simulink model "snap2_f_200msps_64i_4096c"  (R2019a)
settings: Solver=VariableStepDiscrete  StartTime=0.0  StopTime=10.0  RelTol=1e-3
undefined symbols (not defined in the file or in its folder): datetime, posixtime
libraries: xbsIndex_r4 x21354, casper_library_misc x297, casper_library_delays x19, xps_library x14, casper_library_sources x4
(part 40 of 217)

== system snap2_f_200msps_64i_4096c/pfb/pfb16x_0 ==
  note: reshape(reshape([0:8192 - 1], 16, 512)', 1, 8192)
  note: here we get a spectrum
      | 8 channels at a time. It takes
      | 512 clocks to get a full spectrum,
      | then we cycle through 16 inputs
  note: use 32 bit sync
      | because of bug
      | in blackboxing when
      | 1-bit inputs are used
  note: 16 parallel samples on each clock.
      | Consecutive clocks give next 16 samples
      | until all 8k have been sent (taking 512 clocks)
      | Then the block cycles through the different
      | pols
  note: 16 parallel samples on each clock cycle.
      | Consecutive clocks give:
      | pol0
      | pol1
      | ...
      | pol14
      | pol15
  note: Each output here
      | is a consecutive
      | samples for a single ADC
      | input
  note: use 32 bit sync
      | because of bug
      | in blackboxing when
      | 1-bit inputs are used
  sync : Inport
  fft_shift : Inport  Port=2
  din : Inport  Port=3
  stat_rst : Inport  Port=4
  skip_pfb : Inport  Port=5
  Constant : xbsIndex_r4/Constant  const=1.0  gui_display_data_type=Boolean  arith_type=Boolean  n_bits=16  bin_pt=14  preci_type=Single  exp_width=8  frac_width=24  explicit_period=on  period=1  equ=P=C  opselect=C  inp2=PCIN>>17  opr=+  inp1=P  carry=CIN  dbl_ovrd=off  block_type=constant
  Constant1 : xbsIndex_r4/Constant  const=0  gui_display_data_type=Fixed-point  arith_type=Unsigned  n_bits=16  bin_pt=0  preci_type=Single  exp_width=8  frac_width=24  explicit_period=on  period=1  equ=P=C  opselect=C  inp2=PCIN>>17  opr=+  inp1=P  carry=CIN  dbl_ovrd=off  block_type=constant
  Convert{,4..5,7..19} (16 alike) : xbsIndex_r4/Convert  gui_display_data_type=Fixed-point  arith_type="Signed  (2's comp)"  n_bits=18  bin_pt=17  float_type=Single  exp_bits=8  fraction_bits=24  quantization=Truncate  overflow=Wrap  en=off  latency=0  pipeline=off  dbl_ovrd=off  block_type=convert
  Convert1 : xbsIndex_r4/Convert  gui_display_data_type=Boolean  arith_type=Boolean  n_bits=16  bin_pt=0  float_type=Single  exp_bits=8  fraction_bits=24  quantization=Truncate  overflow=Wrap  en=off  latency=0  pipeline=off  dbl_ovrd=off  block_type=convert
  Convert2 : xbsIndex_r4/Convert  gui_display_data_type=Fixed-point  arith_type=Unsigned  n_bits=32  bin_pt=0  float_type=Single  exp_bits=8  fraction_bits=24  quantization=Truncate  overflow=Wrap  en=off  latency=0  pipeline=off  dbl_ovrd=off  block_type=convert
  Convert3 : xbsIndex_r4/Convert  gui_display_data_type=Boolean  arith_type=Boolean  n_bits=16  bin_pt=0  float_type=Single  exp_bits=8  fraction_bits=24  quantization=Truncate  overflow=Wrap  en=off  latency=0  pipeline=off  dbl_ovrd=off  block_type=convert
  Convert6 : xbsIndex_r4/Convert  gui_display_data_type=Fixed-point  arith_type=Unsigned  n_bits=32  bin_pt=0  float_type=Single  exp_bits=8  fraction_bits=24  quantization=Truncate  overflow=Wrap  en=off  latency=0  pipeline=off  dbl_ovrd=off  block_type=convert
  Delay : xbsIndex_r4/Delay  rst=off  infoeditControl=Selection of Reset will increase slice count due to use of real FFs and instead of SRLs  en=off  latency=1  reg_retiming=off  dbl_ovrd=off  block_type=delay
  Delay1 : xbsIndex_r4/Delay  rst=off  infoeditControl=Selection of Reset will increase slice count due to use of real FFs and instead of SRLs  en=off  latency=1  reg_retiming=off  dbl_ovrd=off  block_type=delay
  Mux : xbsIndex_r4/Mux  inputs=2  en=off  latency=1  precision=Full  arith_type=Unsigned  n_bits=16  bin_pt=14  quantization=Truncate  overflow=Wrap  dbl_ovrd=off  block_type=mux
  Mux1 : xbsIndex_r4/Mux  inputs=2  en=off  latency=1  precision=Full  arith_type=Unsigned  n_bits=16  bin_pt=14  quantization=Truncate  overflow=Wrap  dbl_ovrd=off  block_type=mux
  Relational : xbsIndex_r4/Relational  mode=a!=b  op_type=Bool  en=off  latency=1  dbl_ovrd=off  block_type=relational
  bus_create : Subsystem  AncestorBlock=casper_library_flow_control/bus_create  mask(bus_create){inputNum=16}
      mask prompts: inputNum "Number of inputs:"
      mask init:
      | bus_create_init(gcb,...
      |     'inputNum', inputNum);
  bus_create2 : Subsystem  AncestorBlock=casper_library_flow_control/bus_create  mask(bus_create){inputNum=16}
      mask prompts: inputNum "Number of inputs:"
      mask init:
      | bus_create_init(gcb,...
      |     'inputNum', inputNum);
  bus_expand : Subsystem  AncestorBlock=casper_library_flow_control/bus_expand  mask(bus_expand){mode=divisions of equal size, outputNum=16, outputWidth=10, outputBinaryPt=9, outputArithmeticType=1, show_format=off, outputToWorkspace=off, variablePrefix=out, outputToModelAsWell=on}
      mask prompts: outputNum "Number of outputs:"; outputWidth "Output width:"; outputBinaryPt "Output binary point position:"; outputArithmeticType "Output arithmetic type (ufix=0, fix=1, bool=2):"; show_format "Print format string?"; outputToWorkspace "Output to workspace?"; variablePrefix "Variable name prefix:"; outputToModelAsWell "Output to model as well?"
      mask help:
      | Expands a 'bus' made using a bus_create or Xilinx
      | concat block.
      | The input will be divided into the specified number
      | of outputs with the specified arithmetic types.
      | Divisions are made from most significant bit.
      mask init: same as snap2_f_200msps_64i_4096c/autocorr/bus_expand
      settings: AttributesFormatString=16 outputs
      mask TypeOptions mode: divisions of equal size | divisions of arbitrary size
      mask Callback mode: bus_expand_callback();
      mask Callback outputWidth: bus_expand_callback();
      mask Callback outputToWorkspace: bus_expand_callback();
  bus_expand4 : Subsystem  AncestorBlock=casper_library_flow_control/bus_expand  mask(bus_expand){mode=divisions of equal size, outputNum=16, outputWidth=10, outputBinaryPt=0, outputArithmeticType=0, show_format=off, outputToWorkspace=off, variablePrefix=out, outputToModelAsWell=on}
      mask prompts: outputNum "Number of outputs:"; outputWidth "Output width:"; outputBinaryPt "Output binary point position:"; outputArithmeticType "Output arithmetic type (ufix=0, fix=1, bool=2):"; show_format "Print format string?"; outputToWorkspace "Output to workspace?"; variablePrefix "Variable name prefix:"; outputToModelAsWell "Output to model as well?"
      mask help:
      | Expands a 'bus' made using a bus_create or Xilinx
      | concat block.
      | The input will be divided into the specified number
      | of outputs with the specified arithmetic types.
      | Divisions are made from most significant bit.
      mask init: same as snap2_f_200msps_64i_4096c/autocorr/bus_expand
      settings: AttributesFormatString=16 outputs
      mask TypeOptions mode: divisions of equal size | divisions of arbitrary size
      mask Callback mode: bus_expand_callback();
      mask Callback outputWidth: bus_expand_callback();
      mask Callback outputToWorkspace: bus_expand_callback();
  fft_4096_1i : xbsIndex_r4/Black Box  init_code=fft_4096c_1i_core_config  sim_method=Inactive  verbose=off  block_type=blackbox2
  of_count : xbsIndex_r4/Counter  cnt_type=Free Running  cnt_to=Inf  operation=Up  start_count=0  cnt_by_val=1  arith_type=Unsigned  n_bits=32  bin_pt=0  load_pin=off  rst=on  en=on  explicit_period=on  period=1  use_behavioral_HDL=off  implementation=DSP48  dbl_ovrd=off  block_type=counter
  pfb_fir_4096ch_bb : xbsIndex_r4/Black Box  init_code=pfb_fir_4096c_16i_core_config  sim_method=Inactive  verbose=off  block_type=blackbox2
  reorder1 : Subsystem  AncestorBlock=casper_library_reorder/reorder  mask(reorder){map=reshape(reshape([0:8192 - 1], 16, 512)', 1, 8192), n_bits=160, n_inputs=1, bram_latency=2, map_latency=2, fanout_latency=0, double_buffer=0, bram_map=on, software_controlled=off}
      mask prompts: map "Output Order:"; n_bits "Data width in"; n_inputs "Number of inputs"; bram_latency "BRAM Latency"; map_latency "Map Latency"; fanout_latency "Fanout latency"; double_buffer "Double Buffer"; bram_map "Use BlockRAM for Map"; software_controlled "Use runtime software control"
      mask init: same as snap2_f_200msps_64i_4096c/chan_reorder/dynamic
      settings: AttributesFormatString=order=13
      mask Help: eval('xlWeb(''http://casper.berkeley.edu/wiki/Reorder'')')
  square_transposer : Subsystem  AncestorBlock=casper_library_reorder/square_transposer  mask(square_transposer){n_inputs=4, async=off}
      mask prompts: n_inputs "Number of inputs (2^?):"; async "Aynchronus operation"
      mask init:
      | square_transposer_init(gcb,...
      |     'n_inputs', n_inputs, ...
      |     'async', async);
      settings: AttributesFormatString=n_inputs=4
      mask Help: eval('xlWeb(''http://casper.berkeley.edu/wiki/Square_transposer'')')
  status : Subsystem  Tag=xps:sw_reg  AncestorBlock=xps_library/Memory/software_register  mask(swreg){io_dir=To Processor, io_delay=0, init_val=0, sample_period=1, names=reg, bitwidths=32, bin_pts=0, arith_types=0, sim_port=on, show_format=off, desc_str=|}
      mask desc_str=|
      | A 32-bit counter which, for register name suffix
      | ``<n>_status`` increments every time an FFT
      | overflow event is detected in any of FFT channels
      | ``16n..16(n+1)-1``. Resets only when
      | commanded via the PFB control register, and will
      | wrap once the maximum value is reached.
      mask prompts: io_dir "I/O direction"; io_delay "I/O delay"; init_val "Initial Value"; sample_period "Sample period"; names "Bitfield names [msb...lsb]"; bitwidths "Bitfield widths"; bin_pts "Bitfield binary pts"; arith_types "Bitfield types, ufix=0, fix=1, bool=2"; sim_port "Provide sim input/output?"; show_format "Print format string?"; desc_str "Description"
      mask help: A 32-bit software-accessible register. Can be divided into bitfields of varying widths and types using the fields in the block mask.
      mask init:
      | swreg_init(gcb)
      settings: AttributesFormatString=1output
      mask TypeOptions io_dir: To Processor | From Processor
      mask Callback io_dir:
      | mask_enables = get_param(gcb, 'MaskEnables');
      | mask_names = get_param(gcb, 'MaskNames');
      | if strcmp(get_param(gcb, 'io_dir'), 'To Processor'),
      |     mask_enables{ismember(mask_names, 'sample_period')} = 'off';
      | else
      |     mask_enables{ismember(mask_names, 'sample_period')} = 'on';
      | end
      | set_param(gcb, 'MaskEnables', mask_enables);
      mask DialogControl ParameterTabVar0 Prompt: Setup
  sync_out : Outport
  dout : Outport  Port=2
  wires:
  bus_expand4/3(out14) -> square_transposer/4(in2)
  square_transposer/12(out10) -> bus_create2/11(in11)
  bus_expand4/16(lsb_out1) -> square_transposer/17(in15)
  bus_expand4/4(out13) -> square_transposer/5(in3)
  square_transposer/2(out0) -> bus_create2/1(in1)
  square_transposer/13(out11) -> bus_create2/12(in12)
  square_transposer/5(out3) -> bus_create2/4(in4)
  bus_expand4/2(out15) -> square_transposer/3(in1)
  square_transposer/16(out14) -> bus_create2/15(in15)
  bus_expand4/9(out8) -> square_transposer/10(in8)
  square_transposer/10(out8) -> bus_create2/9(in9)
  square_transposer/3(out1) -> bus_create2/2(in2)
  square_transposer/4(out2) -> bus_create2/3(in3)
  bus_expand4/8(out9) -> square_transposer/9(in7)
  square_transposer/15(out13) -> bus_create2/14(in14)
  bus_expand4/10(out7) -> square_transposer/11(in9)
  square_transposer/8(out6) -> bus_create2/7(in7)
  bus_expand4/13(out4) -> square_transposer/14(in12)
  square_transposer/11(out9) -> bus_create2/10(in10)
  bus_expand4/6(out11) -> square_transposer/7(in5)
  square_transposer/14(out12) -> bus_create2/13(in13)
  square_transposer/17(out15) -> bus_create2/16(in16)
  bus_expand4/12(out5) -> square_transposer/13(in11)
  square_transposer/6(out4) -> bus_create2/5(in5)
  square_transposer/7(out5) -> bus_create2/6(in6)
  bus_expand4/14(out3) -> square_transposer/15(in13)
  square_transposer/9(out7) -> bus_create2/8(in8)
  bus_expand4/15(out2) -> square_transposer/16(in14)
  bus_expand4/1(msb_out16) -> square_transposer/2(in0)
  bus_expand4/5(out12) -> square_transposer/6(in4)
  bus_expand4/7(out10) -> square_transposer/8(in6)
  bus_expand4/11(out6) -> square_transposer/12(in10)
  fft_shift/1 -> fft_4096_1i/2
  din/1 -> bus_expand4/1(bus_in)
  pfb_fir_4096ch_bb/1 -> Convert3/1
  fft_4096_1i/1 -> Convert1/1
  fft_4096_1i/2 -> dout/1
  Convert1/1 -> sync_out/1
  Convert2/1 -> pfb_fir_4096ch_bb/1
  Convert6/1 -> fft_4096_1i/1
  fft_4096_1i/3 -> Relational/1
  sync/1 -> square_transposer/1(sync)
  bus_create2/1(bus_out) -> reorder1/3(din0)
  square_transposer/1(sync_out) -> reorder1/1(sync)
  Constant/1 -> reorder1/2(en)
  reorder1/1(sync_out) -> Mux1/3, Convert2/1
  reorder1/3(dout0) -> pfb_fir_4096ch_bb/2, bus_expand/1(bus_in)
  of_count/1 -> status/1(out_reg)
  Constant1/1 -> Relational/2
  Relational/1 -> of_count/2
  stat_rst/1 -> of_count/1
  bus_expand/1(msb_out16) -> Convert/1
  bus_expand/3(out14) -> Convert5/1
  bus_expand/2(out15) -> Convert4/1
  bus_expand/4(out13) -> Convert7/1
  bus_expand/8(out9) -> Convert11/1
  bus_expand/6(out11) -> Convert9/1
  bus_expand/7(out10) -> Convert10/1
  bus_expand/5(out12) -> Convert8/1
  bus_expand/13(out4) -> Convert18/1
  bus_expand/15(out2) -> Convert13/1
  bus_expand/14(out3) -> Convert19/1
  bus_expand/16(lsb_out1) -> Convert14/1
  bus_expand/12(out5) -> Convert17/1
  bus_expand/10(out7) -> Convert15/1
  bus_expand/11(out6) -> Convert16/1
  bus_expand/9(out8) -> Convert12/1
  Convert/1 -> bus_create/1(in1)
  Convert4/1 -> bus_create/2(in2)
  Convert5/1 -> bus_create/3(in3)
  Convert7/1 -> bus_create/4(in4)
  Convert8/1 -> bus_create/5(in5)
  Convert9/1 -> bus_create/6(in6)
  Convert10/1 -> bus_create/7(in7)
  Convert11/1 -> bus_create/8(in8)
  Convert12/1 -> bus_create/9(in9)
  Convert15/1 -> bus_create/10(in10)
  Convert16/1 -> bus_create/11(in11)
  Convert17/1 -> bus_create/12(in12)
  Convert18/1 -> bus_create/13(in13)
  Convert19/1 -> bus_create/14(in14)
  Convert13/1 -> bus_create/15(in15)
  Convert14/1 -> bus_create/16(in16)
  pfb_fir_4096ch_bb/2 -> Mux/2
  bus_create/1(bus_out) -> Mux/3
  Delay/1 -> Mux/1
  Delay1/1 -> Mux1/1
  Convert3/1 -> Mux1/2
  skip_pfb/1 -> Delay/1, Delay1/1
  Mux1/1 -> Convert6/1
  Mux/1 -> fft_4096_1i/3

== system snap2_f_200msps_64i_4096c/pfb/pfb16x_1 ==
  note: use 32 bit sync
      | because of bug
      | in blackboxing when
      | 1-bit inputs are used
  note: Each output here
      | is a consecutive
      | samples for a single ADC
      | input
  note: 16 parallel samples on each clock cycle.
      | Consecutive clocks give:
      | pol0
      | pol1
      | ...
      | pol14
      | pol15
  note: 16 parallel samples on each clock.
      | Consecutive clocks give next 16 samples
      | until all 8k have been sent (taking 512 clocks)
      | Then the block cycles through the different
      | pols
  note: use 32 bit sync
      | because of bug
      | in blackboxing when
      | 1-bit inputs are used
  note: here we get a spectrum
      | 8 channels at a time. It takes
      | 512 clocks to get a full spectrum,
      | then we cycle through 16 inputs
  note: reshape(reshape([0:8192 - 1], 16, 512)', 1, 8192)
  sync : Inport
  fft_shift : Inport  Port=2
  din : Inport  Port=3
  stat_rst : Inport  Port=4
  skip_pfb : Inport  Port=5
  Constant : xbsIndex_r4/Constant  const=1.0  gui_display_data_type=Boolean  arith_type=Boolean  n_bits=16  bin_pt=14  preci_type=Single  exp_width=8  frac_width=24  explicit_period=on  period=1  equ=P=C  opselect=C  inp2=PCIN>>17  opr=+  inp1=P  carry=CIN  dbl_ovrd=off  block_type=constant
  Constant1 : xbsIndex_r4/Constant  const=0  gui_display_data_type=Fixed-point  arith_type=Unsigned  n_bits=16  bin_pt=0  preci_type=Single  exp_width=8  frac_width=24  explicit_period=on  period=1  equ=P=C  opselect=C  inp2=PCIN>>17  opr=+  inp1=P  carry=CIN  dbl_ovrd=off  block_type=constant
  Convert{,4..5,7..19} (16 alike) : xbsIndex_r4/Convert  gui_display_data_type=Fixed-point  arith_type="Signed  (2's comp)"  n_bits=18  bin_pt=17  float_type=Single  exp_bits=8  fraction_bits=24  quantization=Truncate  overflow=Wrap  en=off  latency=0  pipeline=off  dbl_ovrd=off  block_type=convert
  Convert1 : xbsIndex_r4/Convert  gui_display_data_type=Boolean  arith_type=Boolean  n_bits=16  bin_pt=0  float_type=Single  exp_bits=8  fraction_bits=24  quantization=Truncate  overflow=Wrap  en=off  latency=0  pipeline=off  dbl_ovrd=off  block_type=convert
  Convert2 : xbsIndex_r4/Convert  gui_display_data_type=Fixed-point  arith_type=Unsigned  n_bits=32  bin_pt=0  float_type=Single  exp_bits=8  fraction_bits=24  quantization=Truncate  overflow=Wrap  en=off  latency=0  pipeline=off  dbl_ovrd=off  block_type=convert
  Convert3 : xbsIndex_r4/Convert  gui_display_data_type=Boolean  arith_type=Boolean  n_bits=16  bin_pt=0  float_type=Single  exp_bits=8  fraction_bits=24  quantization=Truncate  overflow=Wrap  en=off  latency=0  pipeline=off  dbl_ovrd=off  block_type=convert
  Convert6 : xbsIndex_r4/Convert  gui_display_data_type=Fixed-point  arith_type=Unsigned  n_bits=32  bin_pt=0  float_type=Single  exp_bits=8  fraction_bits=24  quantization=Truncate  overflow=Wrap  en=off  latency=0  pipeline=off  dbl_ovrd=off  block_type=convert
  Delay : xbsIndex_r4/Delay  rst=off  infoeditControl=Selection of Reset will increase slice count due to use of real FFs and instead of SRLs  en=off  latency=1  reg_retiming=off  dbl_ovrd=off  block_type=delay
  Delay1 : xbsIndex_r4/Delay  rst=off  infoeditControl=Selection of Reset will increase slice count due to use of real FFs and instead of SRLs  en=off  latency=1  reg_retiming=off  dbl_ovrd=off  block_type=delay
  Mux : xbsIndex_r4/Mux  inputs=2  en=off  latency=1  precision=Full  arith_type=Unsigned  n_bits=16  bin_pt=14  quantization=Truncate  overflow=Wrap  dbl_ovrd=off  block_type=mux
  Mux1 : xbsIndex_r4/Mux  inputs=2  en=off  latency=1  precision=Full  arith_type=Unsigned  n_bits=16  bin_pt=14  quantization=Truncate  overflow=Wrap  dbl_ovrd=off  block_type=mux
  Relational : xbsIndex_r4/Relational  mode=a!=b  op_type=Bool  en=off  latency=1  dbl_ovrd=off  block_type=relational
  bus_create : Subsystem  AncestorBlock=casper_library_flow_control/bus_create  mask(bus_create){inputNum=16}
      mask prompts: inputNum "Number of inputs:"
      mask init:
      | bus_create_init(gcb,...
      |     'inputNum', inputNum);
  bus_create2 : Subsystem  AncestorBlock=casper_library_flow_control/bus_create  mask(bus_create){inputNum=16}
      mask prompts: inputNum "Number of inputs:"
      mask init:
      | bus_create_init(gcb,...
      |     'inputNum', inputNum);
  bus_expand : Subsystem  AncestorBlock=casper_library_flow_control/bus_expand  mask(bus_expand){mode=divisions of equal size, outputNum=16, outputWidth=10, outputBinaryPt=9, outputArithmeticType=1, show_format=off, outputToWorkspace=off, variablePrefix=out, outputToModelAsWell=on}
      mask prompts: outputNum "Number of outputs:"; outputWidth "Output width:"; outputBinaryPt "Output binary point position:"; outputArithmeticType "Output arithmetic type (ufix=0, fix=1, bool=2):"; show_format "Print format string?"; outputToWorkspace "Output to workspace?"; variablePrefix "Variable name prefix:"; outputToModelAsWell "Output to model as well?"
      mask help:
      | Expands a 'bus' made using a bus_create or Xilinx
      | concat block.
      | The input will be divided into the specified number
      | of outputs with the specified arithmetic types.
      | Divisions are made from most significant bit.
      mask init: same as snap2_f_200msps_64i_4096c/autocorr/bus_expand
      settings: AttributesFormatString=16 outputs
      mask TypeOptions mode: divisions of equal size | divisions of arbitrary size
      mask Callback mode: bus_expand_callback();
      mask Callback outputWidth: bus_expand_callback();
      mask Callback outputToWorkspace: bus_expand_callback();
  bus_expand4 : Subsystem  AncestorBlock=casper_library_flow_control/bus_expand  mask(bus_expand){mode=divisions of equal size, outputNum=16, outputWidth=10, outputBinaryPt=0, outputArithmeticType=0, show_format=off, outputToWorkspace=off, variablePrefix=out, outputToModelAsWell=on}
      mask prompts: outputNum "Number of outputs:"; outputWidth "Output width:"; outputBinaryPt "Output binary point position:"; outputArithmeticType "Output arithmetic type (ufix=0, fix=1, bool=2):"; show_format "Print format string?"; outputToWorkspace "Output to workspace?"; variablePrefix "Variable name prefix:"; outputToModelAsWell "Output to model as well?"
      mask help:
      | Expands a 'bus' made using a bus_create or Xilinx
      | concat block.
      | The input will be divided into the specified number
      | of outputs with the specified arithmetic types.
      | Divisions are made from most significant bit.
      mask init: same as snap2_f_200msps_64i_4096c/autocorr/bus_expand
      settings: AttributesFormatString=16 outputs
      mask TypeOptions mode: divisions of equal size | divisions of arbitrary size
      mask Callback mode: bus_expand_callback();
      mask Callback outputWidth: bus_expand_callback();
      mask Callback outputToWorkspace: bus_expand_callback();
  fft_4096_1i : xbsIndex_r4/Black Box  init_code=fft_4096c_1i_core_config  sim_method=Inactive  verbose=off  block_type=blackbox2
  of_count : xbsIndex_r4/Counter  cnt_type=Free Running  cnt_to=Inf  operation=Up  start_count=0  cnt_by_val=1  arith_type=Unsigned  n_bits=32  bin_pt=0  load_pin=off  rst=on  en=on  explicit_period=on  period=1  use_behavioral_HDL=off  implementation=DSP48  dbl_ovrd=off  block_type=counter
  pfb_fir_4096ch_bb : xbsIndex_r4/Black Box  init_code=pfb_fir_4096c_16i_core_config  sim_method=Inactive  verbose=off  block_type=blackbox2
  reorder1 : Subsystem  AncestorBlock=casper_library_reorder/reorder  mask(reorder){map=reshape(reshape([0:8192 - 1], 16, 512)', 1, 8192), n_bits=160, n_inputs=1, bram_latency=2, map_latency=2, fanout_latency=0, double_buffer=0, bram_map=on, software_controlled=off}
      mask prompts: map "Output Order:"; n_bits "Data width in"; n_inputs "Number of inputs"; bram_latency "BRAM Latency"; map_latency "Map Latency"; fanout_latency "Fanout latency"; double_buffer "Double Buffer"; bram_map "Use BlockRAM for Map"; software_controlled "Use runtime software control"
      mask init: same as snap2_f_200msps_64i_4096c/chan_reorder/dynamic
      settings: AttributesFormatString=order=13
      mask Help: eval('xlWeb(''http://casper.berkeley.edu/wiki/Reorder'')')
  square_transposer : Subsystem  AncestorBlock=casper_library_reorder/square_transposer  mask(square_transposer){n_inputs=4, async=off}
      mask prompts: n_inputs "Number of inputs (2^?):"; async "Aynchronus operation"
      mask init:
      | square_transposer_init(gcb,...
      |     'n_inputs', n_inputs, ...
      |     'async', async);
      settings: AttributesFormatString=n_inputs=4
      mask Help: eval('xlWeb(''http://casper.berkeley.edu/wiki/Square_transposer'')')
  status : Subsystem  Tag=xps:sw_reg  AncestorBlock=xps_library/Memory/software_register  mask(swreg){io_dir=To Processor, io_delay=0, init_val=0, sample_period=1, names=reg, bitwidths=32, bin_pts=0, arith_types=0, sim_port=on, show_format=off, desc_str=|}
      mask desc_str=|
      | A 32-bit counter which, for register name suffix
      | ``<n>_status`` increments every time an FFT
      | overflow event is detected in any of FFT channels
      | ``16n..16(n+1)-1``. Resets only when
      | commanded via the PFB control register, and will
      | wrap once the maximum value is reached.
      mask prompts: io_dir "I/O direction"; io_delay "I/O delay"; init_val "Initial Value"; sample_period "Sample period"; names "Bitfield names [msb...lsb]"; bitwidths "Bitfield widths"; bin_pts "Bitfield binary pts"; arith_types "Bitfield types, ufix=0, fix=1, bool=2"; sim_port "Provide sim input/output?"; show_format "Print format string?"; desc_str "Description"
      mask help: A 32-bit software-accessible register. Can be divided into bitfields of varying widths and types using the fields in the block mask.
      mask init:
      | swreg_init(gcb)
      settings: AttributesFormatString=1output
      mask TypeOptions io_dir: To Processor | From Processor
      mask Callback io_dir:
      | mask_enables = get_param(gcb, 'MaskEnables');
      | mask_names = get_param(gcb, 'MaskNames');
      | if strcmp(get_param(gcb, 'io_dir'), 'To Processor'),
      |     mask_enables{ismember(mask_names, 'sample_period')} = 'off';
      | else
      |     mask_enables{ismember(mask_names, 'sample_period')} = 'on';
      | end
      | set_param(gcb, 'MaskEnables', mask_enables);
      mask DialogControl ParameterTabVar0 Prompt: Setup
  sync_out : Outport
  dout : Outport  Port=2
  wires:
  Mux/1 -> fft_4096_1i/3
  Mux1/1 -> Convert6/1
  skip_pfb/1 -> Delay1/1, Delay/1
  Convert3/1 -> Mux1/2
  Delay1/1 -> Mux1/1
  Delay/1 -> Mux/1
  bus_create/1(bus_out) -> Mux/3
  pfb_fir_4096ch_bb/2 -> Mux/2
  Convert14/1 -> bus_create/16(in16)
  Convert13/1 -> bus_create/15(in15)
  Convert19/1 -> bus_create/14(in14)
  Convert18/1 -> bus_create/13(in13)
  Convert17/1 -> bus_create/12(in12)
  Convert16/1 -> bus_create/11(in11)
  Convert15/1 -> bus_create/10(in10)
  Convert12/1 -> bus_create/9(in9)
  Convert11/1 -> bus_create/8(in8)
  Convert10/1 -> bus_create/7(in7)
  Convert9/1 -> bus_create/6(in6)
  Convert8/1 -> bus_create/5(in5)
  Convert7/1 -> bus_create/4(in4)
  Convert5/1 -> bus_create/3(in3)
  Convert4/1 -> bus_create/2(in2)
  Convert/1 -> bus_create/1(in1)
  bus_expand/9(out8) -> Convert12/1
  bus_expand/11(out6) -> Convert16/1
  bus_expand/10(out7) -> Convert15/1
  bus_expand/12(out5) -> Convert17/1
  bus_expand/16(lsb_out1) -> Convert14/1
  bus_expand/14(out3) -> Convert19/1
  bus_expand/15(out2) -> Convert13/1
  bus_expand/13(out4) -> Convert18/1
  bus_expand/5(out12) -> Convert8/1
  bus_expand/7(out10) -> Convert10/1
  bus_expand/6(out11) -> Convert9/1
  bus_expand/8(out9) -> Convert11/1
  bus_expand/4(out13) -> Convert7/1
  bus_expand/2(out15) -> Convert4/1
  bus_expand/3(out14) -> Convert5/1
  bus_expand/1(msb_out16) -> Convert/1
  stat_rst/1 -> of_count/1
  Relational/1 -> of_count/2
  Constant1/1 -> Relational/2
  of_count/1 -> status/1(out_reg)
  reorder1/3(dout0) -> bus_expand/1(bus_in), pfb_fir_4096ch_bb/2
  reorder1/1(sync_out) -> Convert2/1, Mux1/3
  Constant/1 -> reorder1/2(en)
  square_transposer/1(sync_out) -> reorder1/1(sync)
  bus_create2/1(bus_out) -> reorder1/3(din0)
  sync/1 -> square_transposer/1(sync)
  fft_4096_1i/3 -> Relational/1
  Convert6/1 -> fft_4096_1i/1
  Convert2/1 -> pfb_fir_4096ch_bb/1
  Convert1/1 -> sync_out/1
  fft_4096_1i/2 -> dout/1
  fft_4096_1i/1 -> Convert1/1
  pfb_fir_4096ch_bb/1 -> Convert3/1
  din/1 -> bus_expand4/1(bus_in)
  fft_shift/1 -> fft_4096_1i/2
  bus_expand4/11(out6) -> square_transposer/12(in10)
  bus_expand4/7(out10) -> square_transposer/8(in6)
  bus_expand4/5(out12) -> square_transposer/6(in4)
  bus_expand4/1(msb_out16) -> square_transposer/2(in0)
  bus_expand4/15(out2) -> square_transposer/16(in14)
  square_transposer/9(out7) -> bus_create2/8(in8)
  bus_expand4/14(out3) -> square_transposer/15(in13)
  square_transposer/7(out5) -> bus_create2/6(in6)
  square_transposer/6(out4) -> bus_create2/5(in5)
  bus_expand4/12(out5) -> square_transposer/13(in11)
  square_transposer/17(out15) -> bus_create2/16(in16)
  square_transposer/14(out12) -> bus_create2/13(in13)
  bus_expand4/6(out11) -> square_transposer/7(in5)
  square_transposer/11(out9) -> bus_create2/10(in10)
  bus_expand4/13(out4) -> square_transposer/14(in12)
  square_transposer/8(out6) -> bus_create2/7(in7)
  bus_expand4/10(out7) -> square_transposer/11(in9)
  square_transposer/15(out13) -> bus_create2/14(in14)
  bus_expand4/8(out9) -> square_transposer/9(in7)
  square_transposer/4(out2) -> bus_create2/3(in3)
  square_transposer/3(out1) -> bus_create2/2(in2)
  square_transposer/10(out8) -> bus_create2/9(in9)
  bus_expand4/9(out8) -> square_transposer/10(in8)
  square_transposer/16(out14) -> bus_create2/15(in15)
  bus_expand4/2(out15) -> square_transposer/3(in1)
  square_transposer/5(out3) -> bus_create2/4(in4)
  square_transposer/13(out11) -> bus_create2/12(in12)
  square_transposer/2(out0) -> bus_create2/1(in1)
  bus_expand4/4(out13) -> square_transposer/5(in3)
  bus_expand4/16(lsb_out1) -> square_transposer/17(in15)
  square_transposer/12(out10) -> bus_create2/11(in11)
  bus_expand4/3(out14) -> square_transposer/4(in2)

== system snap2_f_200msps_64i_4096c/pfb/pfb16x_2 ==
  note: reshape(reshape([0:8192 - 1], 16, 512)', 1, 8192)
  note: here we get a spectrum
      | 8 channels at a time. It takes
      | 512 clocks to get a full spectrum,
      | then we cycle through 16 inputs
  note: use 32 bit sync
      | because of bug
      | in blackboxing when
      | 1-bit inputs are used
  note: 16 parallel samples on each clock.
      | Consecutive clocks give next 16 samples
      | until all 8k have been sent (taking 512 clocks)
      | Then the block cycles through the different
      | pols
  note: 16 parallel samples on each clock cycle.
      | Consecutive clocks give:
      | pol0
      | pol1
      | ...
      | pol14
      | pol15
  note: Each output here
      | is a consecutive
      | samples for a single ADC
      | input
  note: use 32 bit sync
      | because of bug
      | in blackboxing when
      | 1-bit inputs are used
  sync : Inport
  fft_shift : Inport  Port=2
  din : Inport  Port=3
  stat_rst : Inport  Port=4
  skip_pfb : Inport  Port=5
  Constant : xbsIndex_r4/Constant  const=1.0  gui_display_data_type=Boolean  arith_type=Boolean  n_bits=16  bin_pt=14  preci_type=Single  exp_width=8  frac_width=24  explicit_period=on  period=1  equ=P=C  opselect=C  inp2=PCIN>>17  opr=+  inp1=P  carry=CIN  dbl_ovrd=off  block_type=constant
  Constant1 : xbsIndex_r4/Constant  const=0  gui_display_data_type=Fixed-point  arith_type=Unsigned  n_bits=16  bin_pt=0  preci_type=Single  exp_width=8  frac_width=24  explicit_period=on  period=1  equ=P=C  opselect=C  inp2=PCIN>>17  opr=+  inp1=P  carry=CIN  dbl_ovrd=off  block_type=constant
  Convert{,4..5,7..19} (16 alike) : xbsIndex_r4/Convert  gui_display_data_type=Fixed-point  arith_type="Signed  (2's comp)"  n_bits=18  bin_pt=17  float_type=Single  exp_bits=8  fraction_bits=24  quantization=Truncate  overflow=Wrap  en=off  latency=0  pipeline=off  dbl_ovrd=off  block_type=convert
  Convert1 : xbsIndex_r4/Convert  gui_display_data_type=Boolean  arith_type=Boolean  n_bits=16  bin_pt=0  float_type=Single  exp_bits=8  fraction_bits=24  quantization=Truncate  overflow=Wrap  en=off  latency=0  pipeline=off  dbl_ovrd=off  block_type=convert
  Convert2 : xbsIndex_r4/Convert  gui_display_data_type=Fixed-point  arith_type=Unsigned  n_bits=32  bin_pt=0  float_type=Single  exp_bits=8  fraction_bits=24  quantization=Truncate  overflow=Wrap  en=off  latency=0  pipeline=off  dbl_ovrd=off  block_type=convert
  Convert3 : xbsIndex_r4/Convert  gui_display_data_type=Boolean  arith_type=Boolean  n_bits=16  bin_pt=0  float_type=Single  exp_bits=8  fraction_bits=24  quantization=Truncate  overflow=Wrap  en=off  latency=0  pipeline=off  dbl_ovrd=off  block_type=convert
  Convert6 : xbsIndex_r4/Convert  gui_display_data_type=Fixed-point  arith_type=Unsigned  n_bits=32  bin_pt=0  float_type=Single  exp_bits=8  fraction_bits=24  quantization=Truncate  overflow=Wrap  en=off  latency=0  pipeline=off  dbl_ovrd=off  block_type=convert
  Delay : xbsIndex_r4/Delay  rst=off  infoeditControl=Selection of Reset will increase slice count due to use of real FFs and instead of SRLs  en=off  latency=1  reg_retiming=off  dbl_ovrd=off  block_type=delay
  Delay1 : xbsIndex_r4/Delay  rst=off  infoeditControl=Selection of Reset will increase slice count due to use of real FFs and instead of SRLs  en=off  latency=1  reg_retiming=off  dbl_ovrd=off  block_type=delay
  Mux : xbsIndex_r4/Mux  inputs=2  en=off  latency=1  precision=Full  arith_type=Unsigned  n_bits=16  bin_pt=14  quantization=Truncate  overflow=Wrap  dbl_ovrd=off  block_type=mux
  Mux1 : xbsIndex_r4/Mux  inputs=2  en=off  latency=1  precision=Full  arith_type=Unsigned  n_bits=16  bin_pt=14  quantization=Truncate  overflow=Wrap  dbl_ovrd=off  block_type=mux
  Relational : xbsIndex_r4/Relational  mode=a!=b  op_type=Bool  en=off  latency=1  dbl_ovrd=off  block_type=relational
  bus_create : Subsystem  AncestorBlock=casper_library_flow_control/bus_create  mask(bus_create){inputNum=16}
      mask prompts: inputNum "Number of inputs:"
      mask init:
      | bus_create_init(gcb,...
      |     'inputNum', inputNum);
  bus_create2 : Subsystem  AncestorBlock=casper_library_flow_control/bus_create  mask(bus_create){inputNum=16}
      mask prompts: inputNum "Number of inputs:"
      mask init:
      | bus_create_init(gcb,...
      |     'inputNum', inputNum);
  bus_expand : Subsystem  AncestorBlock=casper_library_flow_control/bus_expand  mask(bus_expand){mode=divisions of equal size, outputNum=16, outputWidth=10, outputBinaryPt=9, outputArithmeticType=1, show_format=off, outputToWorkspace=off, variablePrefix=out, outputToModelAsWell=on}
      mask prompts: outputNum "Number of outputs:"; outputWidth "Output width:"; outputBinaryPt "Output binary point position:"; outputArithmeticType "Output arithmetic type (ufix=0, fix=1, bool=2):"; show_format "Print format string?"; outputToWorkspace "Output to workspace?"; variablePrefix "Variable name prefix:"; outputToModelAsWell "Output to model as well?"
      mask help:
      | Expands a 'bus' made using a bus_create or Xilinx
      | concat block.
      | The input will be divided into the specified number
      | of outputs with the specified arithmetic types.
      | Divisions are made from most significant bit.
      mask init: same as snap2_f_200msps_64i_4096c/autocorr/bus_expand
      settings: AttributesFormatString=16 outputs
      mask TypeOptions mode: divisions of equal size | divisions of arbitrary size
      mask Callback mode: bus_expand_callback();
      mask Callback outputWidth: bus_expand_callback();
      mask Callback outputToWorkspace: bus_expand_callback();
  bus_expand4 : Subsystem  AncestorBlock=casper_library_flow_control/bus_expand  mask(bus_expand){mode=divisions of equal size, outputNum=16, outputWidth=10, outputBinaryPt=0, outputArithmeticType=0, show_format=off, outputToWorkspace=off, variablePrefix=out, outputToModelAsWell=on}
      mask prompts: outputNum "Number of outputs:"; outputWidth "Output width:"; outputBinaryPt "Output binary point position:"; outputArithmeticType "Output arithmetic type (ufix=0, fix=1, bool=2):"; show_format "Print format string?"; outputToWorkspace "Output to workspace?"; variablePrefix "Variable name prefix:"; outputToModelAsWell "Output to model as well?"
      mask help:
      | Expands a 'bus' made using a bus_create or Xilinx
      | concat block.
      | The input will be divided into the specified number
      | of outputs with the specified arithmetic types.
      | Divisions are made from most significant bit.
      mask init: same as snap2_f_200msps_64i_4096c/autocorr/bus_expand
      settings: AttributesFormatString=16 outputs
      mask TypeOptions mode: divisions of equal size | divisions of arbitrary size
      mask Callback mode: bus_expand_callback();
      mask Callback outputWidth: bus_expand_callback();
      mask Callback outputToWorkspace: bus_expand_callback();
  fft_4096_1i : xbsIndex_r4/Black Box  init_code=fft_4096c_1i_core_config  sim_method=Inactive  verbose=off  block_type=blackbox2
  of_count : xbsIndex_r4/Counter  cnt_type=Free Running  cnt_to=Inf  operation=Up  start_count=0  cnt_by_val=1  arith_type=Unsigned  n_bits=32  bin_pt=0  load_pin=off  rst=on  en=on  explicit_period=on  period=1  use_behavioral_HDL=off  implementation=DSP48  dbl_ovrd=off  block_type=counter
  pfb_fir_4096ch_bb : xbsIndex_r4/Black Box  init_code=pfb_fir_4096c_16i_core_config  sim_method=Inactive  verbose=off  block_type=blackbox2
  reorder1 : Subsystem  AncestorBlock=casper_library_reorder/reorder  mask(reorder){map=reshape(reshape([0:8192 - 1], 16, 512)', 1, 8192), n_bits=160, n_inputs=1, bram_latency=2, map_latency=2, fanout_latency=0, double_buffer=0, bram_map=on, software_controlled=off}
      mask prompts: map "Output Order:"; n_bits "Data width in"; n_inputs "Number of inputs"; bram_latency "BRAM Latency"; map_latency "Map Latency"; fanout_latency "Fanout latency"; double_buffer "Double Buffer"; bram_map "Use BlockRAM for Map"; software_controlled "Use runtime software control"
      mask init: same as snap2_f_200msps_64i_4096c/chan_reorder/dynamic
      settings: AttributesFormatString=order=13
      mask Help: eval('xlWeb(''http://casper.berkeley.edu/wiki/Reorder'')')
  square_transposer : Subsystem  AncestorBlock=casper_library_reorder/square_transposer  mask(square_transposer){n_inputs=4, async=off}
      mask prompts: n_inputs "Number of inputs (2^?):"; async "Aynchronus operation"
      mask init:
      | square_transposer_init(gcb,...
      |     'n_inputs', n_inputs, ...
      |     'async', async);
      settings: AttributesFormatString=n_inputs=4
      mask Help: eval('xlWeb(''http://casper.berkeley.edu/wiki/Square_transposer'')')
  status : Subsystem  Tag=xps:sw_reg  AncestorBlock=xps_library/Memory/software_register  mask(swreg){io_dir=To Processor, io_delay=0, init_val=0, sample_period=1, names=reg, bitwidths=32, bin_pts=0, arith_types=0, sim_port=on, show_format=off, desc_str=|}
      mask desc_str=|
      | A 32-bit counter which, for register name suffix
      | ``<n>_status`` increments every time an FFT
      | overflow event is detected in any of FFT channels
      | ``16n..16(n+1)-1``. Resets only when
      | commanded via the PFB control register, and will
      | wrap once the maximum value is reached.
      mask prompts: io_dir "I/O direction"; io_delay "I/O delay"; init_val "Initial Value"; sample_period "Sample period"; names "Bitfield names [msb...lsb]"; bitwidths "Bitfield widths"; bin_pts "Bitfield binary pts"; arith_types "Bitfield types, ufix=0, fix=1, bool=2"; sim_port "Provide sim input/output?"; show_format "Print format string?"; desc_str "Description"
      mask help: A 32-bit software-accessible register. Can be divided into bitfields of varying widths and types using the fields in the block mask.
      mask init:
      | swreg_init(gcb)
      settings: AttributesFormatString=1output
      mask TypeOptions io_dir: To Processor | From Processor
      mask Callback io_dir:
      | mask_enables = get_param(gcb, 'MaskEnables');
      | mask_names = get_param(gcb, 'MaskNames');
      | if strcmp(get_param(gcb, 'io_dir'), 'To Processor'),
      |     mask_enables{ismember(mask_names, 'sample_period')} = 'off';
      | else
      |     mask_enables{ismember(mask_names, 'sample_period')} = 'on';
      | end
      | set_param(gcb, 'MaskEnables', mask_enables);
      mask DialogControl ParameterTabVar0 Prompt: Setup
  sync_out : Outport
  dout : Outport  Port=2
  wires:
  bus_expand4/3(out14) -> square_transposer/4(in2)
  square_transposer/12(out10) -> bus_create2/11(in11)
  bus_expand4/16(lsb_out1) -> square_transposer/17(in15)
  bus_expand4/4(out13) -> square_transposer/5(in3)
  square_transposer/2(out0) -> bus_create2/1(in1)
  square_transposer/13(out11) -> bus_create2/12(in12)
  square_transposer/5(out3) -> bus_create2/4(in4)
  bus_expand4/2(out15) -> square_transposer/3(in1)
  square_transposer/16(out14) -> bus_create2/15(in15)
  bus_expand4/9(out8) -> square_transposer/10(in8)
  square_transposer/10(out8) -> bus_create2/9(in9)
  square_transposer/3(out1) -> bus_create2/2(in2)
  square_transposer/4(out2) -> bus_create2/3(in3)
  bus_expand4/8(out9) -> square_transposer/9(in7)
  square_transposer/15(out13) -> bus_create2/14(in14)
  bus_expand4/10(out7) -> square_transposer/11(in9)
  square_transposer/8(out6) -> bus_create2/7(in7)
  bus_expand4/13(out4) -> square_transposer/14(in12)
  square_transposer/11(out9) -> bus_create2/10(in10)
  bus_expand4/6(out11) -> square_transposer/7(in5)
  square_transposer/14(out12) -> bus_create2/13(in13)
  square_transposer/17(out15) -> bus_create2/16(in16)
  bus_expand4/12(out5) -> square_transposer/13(in11)
  square_transposer/6(out4) -> bus_create2/5(in5)
  square_transposer/7(out5) -> bus_create2/6(in6)
  bus_expand4/14(out3) -> square_transposer/15(in13)
  square_transposer/9(out7) -> bus_create2/8(in8)
  bus_expand4/15(out2) -> square_transposer/16(in14)
  bus_expand4/1(msb_out16) -> square_transposer/2(in0)
  bus_expand4/5(out12) -> square_transposer/6(in4)
  bus_expand4/7(out10) -> square_transposer/8(in6)
  bus_expand4/11(out6) -> square_transposer/12(in10)
  fft_shift/1 -> fft_4096_1i/2
  din/1 -> bus_expand4/1(bus_in)
  pfb_fir_4096ch_bb/1 -> Convert3/1
  fft_4096_1i/1 -> Convert1/1
  fft_4096_1i/2 -> dout/1
  Convert1/1 -> sync_out/1
  Convert2/1 -> pfb_fir_4096ch_bb/1
  Convert6/1 -> fft_4096_1i/1
  fft_4096_1i/3 -> Relational/1
  sync/1 -> square_transposer/1(sync)
  bus_create2/1(bus_out) -> reorder1/3(din0)
  square_transposer/1(sync_out) -> reorder1/1(sync)
  Constant/1 -> reorder1/2(en)
  reorder1/1(sync_out) -> Mux1/3, Convert2/1
  reorder1/3(dout0) -> pfb_fir_4096ch_bb/2, bus_expand/1(bus_in)
  of_count/1 -> status/1(out_reg)
  Constant1/1 -> Relational/2
  Relational/1 -> of_count/2
  stat_rst/1 -> of_count/1
  bus_expand/1(msb_out16) -> Convert/1
  bus_expand/3(out14) -> Convert5/1
  bus_expand/2(out15) -> Convert4/1
  bus_expand/4(out13) -> Convert7/1
  bus_expand/8(out9) -> Convert11/1
  bus_expand/6(out11) -> Convert9/1
  bus_expand/7(out10) -> Convert10/1
  bus_expand/5(out12) -> Convert8/1
  bus_expand/13(out4) -> Convert18/1
  bus_expand/15(out2) -> Convert13/1
  bus_expand/14(out3) -> Convert19/1
  bus_expand/16(lsb_out1) -> Convert14/1
  bus_expand/12(out5) -> Convert17/1
  bus_expand/10(out7) -> Convert15/1
  bus_expand/11(out6) -> Convert16/1
  bus_expand/9(out8) -> Convert12/1
  Convert/1 -> bus_create/1(in1)
  Convert4/1 -> bus_create/2(in2)
  Convert5/1 -> bus_create/3(in3)
  Convert7/1 -> bus_create/4(in4)
  Convert8/1 -> bus_create/5(in5)
  Convert9/1 -> bus_create/6(in6)
  Convert10/1 -> bus_create/7(in7)
  Convert11/1 -> bus_create/8(in8)
  Convert12/1 -> bus_create/9(in9)
  Convert15/1 -> bus_create/10(in10)
  Convert16/1 -> bus_create/11(in11)
  Convert17/1 -> bus_create/12(in12)
  Convert18/1 -> bus_create/13(in13)
  Convert19/1 -> bus_create/14(in14)
  Convert13/1 -> bus_create/15(in15)
  Convert14/1 -> bus_create/16(in16)
  pfb_fir_4096ch_bb/2 -> Mux/2
  bus_create/1(bus_out) -> Mux/3
  Delay/1 -> Mux/1
  Delay1/1 -> Mux1/1
  Convert3/1 -> Mux1/2
  skip_pfb/1 -> Delay/1, Delay1/1
  Mux1/1 -> Convert6/1
  Mux/1 -> fft_4096_1i/3
